simulink model "PWMGenerator"  (R2017a)
settings: Solver=VariableStepAuto  StartTime=0.0  StopTime=2000000  RelTol=1e-3
libraries: hdlsllib x15, simulink x5
settings Model: Creator=Ryan Corkery  LastModifiedBy=nguyen.se
settings OptimizationCC: BlockReduction=off  ConditionallyExecuteInputs=off  DefaultParameterBehavior=Inlined
settings DebuggingCC: AlgebraicLoopMsg=error
settings HardwareCC: ProdBitPerPointer=32  ProdBitPerSizeT=32  ProdBitPerPtrDiffT=32  ProdLargestAtomicFloat=None  ProdIntDivRoundTo=Undefined  ProdEndianess=Unspecified  ProdWordSize=32  ProdHWDeviceType=ASIC/FPGA->ASIC/FPGA  ProdEqTarget=off

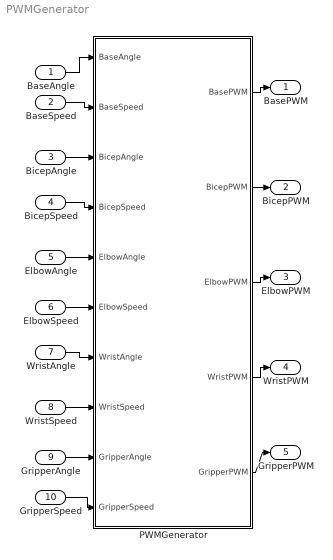
== system PWMGenerator ==
  BaseAngle : Inport  OutDataTypeStr=uint8
  BaseSpeed : Inport  Port=2  OutDataTypeStr=uint8
  BicepAngle : Inport  Port=3  OutDataTypeStr=uint8
  BicepSpeed : Inport  Port=4  OutDataTypeStr=uint8
  ElbowAngle : Inport  Port=5  OutDataTypeStr=uint8
  ElbowSpeed : Inport  Port=6  OutDataTypeStr=uint8
  WristAngle : Inport  Port=7  OutDataTypeStr=uint8
  WristSpeed : Inport  Port=8  OutDataTypeStr=uint8
  GripperAngle : Inport  Port=9  OutDataTypeStr=uint8
  GripperSpeed : Inport  Port=10  OutDataTypeStr=uint8
  PWMGenerator : Subsystem
  BasePWM : Outport  OutDataTypeStr=boolean
  BicepPWM : Outport  Port=2  OutDataTypeStr=boolean
  ElbowPWM : Outport  Port=3  OutDataTypeStr=boolean
  WristPWM : Outport  Port=4  OutDataTypeStr=boolean
  GripperPWM : Outport  Port=5  OutDataTypeStr=boolean
  wires:
  BaseAngle/1 -> PWMGenerator/1(BaseAngle)
  BaseSpeed/1 -> PWMGenerator/2(BaseSpeed)
  BicepAngle/1 -> PWMGenerator/3(BicepAngle)
  BicepSpeed/1 -> PWMGenerator/4(BicepSpeed)
  ElbowAngle/1 -> PWMGenerator/5(ElbowAngle)
  ElbowSpeed/1 -> PWMGenerator/6(ElbowSpeed)
  WristAngle/1 -> PWMGenerator/7(WristAngle)
  WristSpeed/1 -> PWMGenerator/8(WristSpeed)
  GripperAngle/1 -> PWMGenerator/9(GripperAngle)
  GripperSpeed/1 -> PWMGenerator/10(GripperSpeed)
  PWMGenerator/1(BasePWM) -> BasePWM/1
  PWMGenerator/2(BicepPWM) -> BicepPWM/1
  PWMGenerator/3(ElbowPWM) -> ElbowPWM/1
  PWMGenerator/4(WristPWM) -> WristPWM/1
  PWMGenerator/5(GripperPWM) -> GripperPWM/1

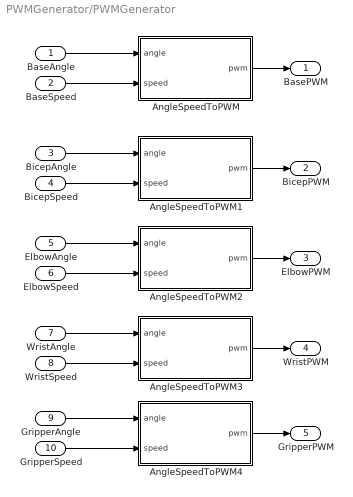
== system PWMGenerator/PWMGenerator ==
  BaseAngle : Inport  OutDataTypeStr=uint8
  BaseSpeed : Inport  Port=2  OutDataTypeStr=uint8
  BicepAngle : Inport  Port=3  OutDataTypeStr=uint8
  BicepSpeed : Inport  Port=4  OutDataTypeStr=uint8
  ElbowAngle : Inport  Port=5  OutDataTypeStr=uint8
  ElbowSpeed : Inport  Port=6  OutDataTypeStr=uint8
  WristAngle : Inport  Port=7  OutDataTypeStr=uint8
  WristSpeed : Inport  Port=8  OutDataTypeStr=uint8
  GripperAngle : Inport  Port=9  OutDataTypeStr=uint8
  GripperSpeed : Inport  Port=10  OutDataTypeStr=uint8
  AngleSpeedToPWM : Subsystem
  AngleSpeedToPWM1 : Subsystem
  AngleSpeedToPWM2 : Subsystem
  AngleSpeedToPWM3 : Subsystem
  AngleSpeedToPWM4 : Subsystem
  BasePWM : Outport  OutDataTypeStr=boolean
  BicepPWM : Outport  Port=2  OutDataTypeStr=boolean
  ElbowPWM : Outport  Port=3  OutDataTypeStr=boolean
  WristPWM : Outport  Port=4  OutDataTypeStr=boolean
  GripperPWM : Outport  Port=5  OutDataTypeStr=boolean
  wires:
  WristAngle/1 -> AngleSpeedToPWM3/1(angle)
  BaseAngle/1 -> AngleSpeedToPWM/1(angle)
  GripperSpeed/1 -> AngleSpeedToPWM4/2("speed ")
  WristSpeed/1 -> AngleSpeedToPWM3/2("speed ")
  GripperAngle/1 -> AngleSpeedToPWM4/1(angle)
  ElbowSpeed/1 -> AngleSpeedToPWM2/2("speed ")
  AngleSpeedToPWM/1(pwm) -> BasePWM/1
  AngleSpeedToPWM1/1(pwm) -> BicepPWM/1
  AngleSpeedToPWM2/1(pwm) -> ElbowPWM/1
  AngleSpeedToPWM3/1(pwm) -> WristPWM/1
  AngleSpeedToPWM4/1(pwm) -> GripperPWM/1
  BicepAngle/1 -> AngleSpeedToPWM1/1(angle)
  ElbowAngle/1 -> AngleSpeedToPWM2/1(angle)
  BicepSpeed/1 -> AngleSpeedToPWM1/2("speed ")
  BaseSpeed/1 -> AngleSpeedToPWM/2("speed ")

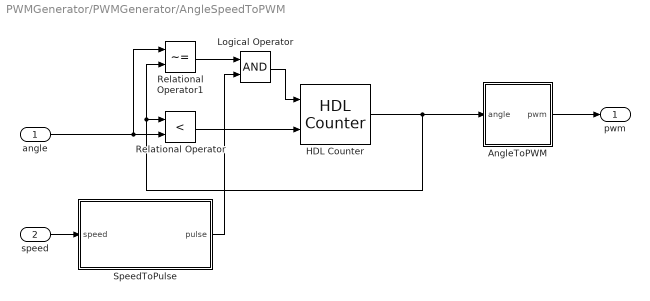
== system PWMGenerator/PWMGenerator/AngleSpeedToPWM ==
  angle : Inport  OutDataTypeStr=uint8
  "speed " : Inport  Port=2  OutDataTypeStr=uint8
  AngleToPWM : Subsystem
  HDL Counter : hdlsllib/HDL Operations/HDL Counter  CountType=Count limited  CountInit=90  CountStep=1  CountMax=180  CountFromType=Specify  CountFrom=0  CountResetPort=off  CountLoadPort=off  CountEnbPort=on  CountDirPort=on  CountDataType=Unsigned  CountWordLen=8  CountFracLen=0  CountSampTime=1
      settings: SourceProductName=HDL Coder  SourceProductBaseCode=HD
  Logical Operator : Logic  AllPortsSameDT=off  OutDataTypeStr=boolean
  Relational Operator : RelationalOperator  Operator=<  OutDataTypeStr=boolean  RndMeth=Simplest
  Relational Operator1 : RelationalOperator  Operator=~=  OutDataTypeStr=boolean  RndMeth=Simplest
  SpeedToPulse : Subsystem
  pwm : Outport  OutDataTypeStr=boolean
  wires:
  Relational Operator1/1 -> Logical Operator/1
  AngleToPWM/1(pwm) -> pwm/1
  HDL Counter/1 -> AngleToPWM/1("angle "), Relational Operator1/2, Relational Operator/1
  SpeedToPulse/1(pulse) -> Logical Operator/2
  Relational Operator/1 -> HDL Counter/2
  angle/1 -> Relational Operator1/1, Relational Operator/2
  Logical Operator/1 -> HDL Counter/1
  "speed "/1 -> SpeedToPulse/1(speed)

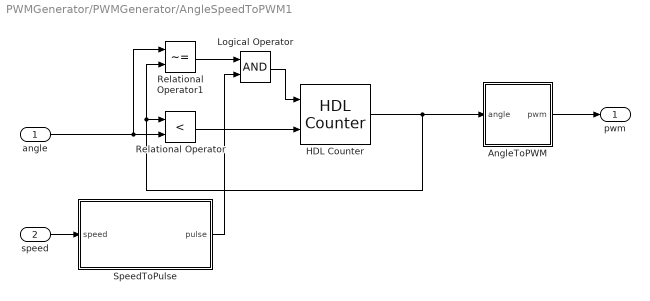
== system PWMGenerator/PWMGenerator/AngleSpeedToPWM1 ==
  angle : Inport  OutDataTypeStr=uint8
  "speed " : Inport  Port=2  OutDataTypeStr=uint8
  AngleToPWM : Subsystem
  HDL Counter : hdlsllib/HDL Operations/HDL Counter  CountType=Count limited  CountInit=90  CountStep=1  CountMax=180  CountFromType=Specify  CountFrom=0  CountResetPort=off  CountLoadPort=off  CountEnbPort=on  CountDirPort=on  CountDataType=Unsigned  CountWordLen=8  CountFracLen=0  CountSampTime=1
      settings: SourceProductName=HDL Coder  SourceProductBaseCode=HD
  Logical Operator : Logic  AllPortsSameDT=off  OutDataTypeStr=boolean
  Relational Operator : RelationalOperator  Operator=<  OutDataTypeStr=boolean  RndMeth=Simplest
  Relational Operator1 : RelationalOperator  Operator=~=  OutDataTypeStr=boolean  RndMeth=Simplest
  SpeedToPulse : Subsystem
  pwm : Outport  OutDataTypeStr=boolean
  wires:
  Relational Operator1/1 -> Logical Operator/1
  AngleToPWM/1(pwm) -> pwm/1
  HDL Counter/1 -> AngleToPWM/1("angle "), Relational Operator1/2, Relational Operator/1
  SpeedToPulse/1(pulse) -> Logical Operator/2
  Relational Operator/1 -> HDL Counter/2
  angle/1 -> Relational Operator1/1, Relational Operator/2
  Logical Operator/1 -> HDL Counter/1
  "speed "/1 -> SpeedToPulse/1(speed)

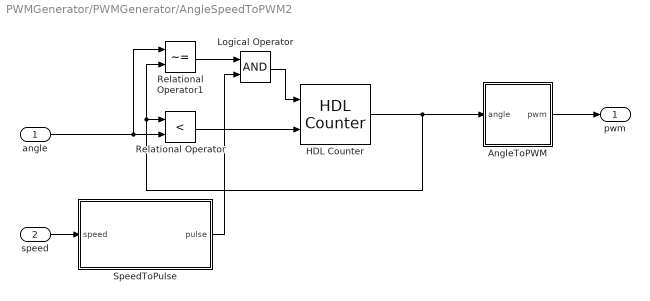
== system PWMGenerator/PWMGenerator/AngleSpeedToPWM2 ==
  angle : Inport  OutDataTypeStr=uint8
  "speed " : Inport  Port=2  OutDataTypeStr=uint8
  AngleToPWM : Subsystem
  HDL Counter : hdlsllib/HDL Operations/HDL Counter  CountType=Count limited  CountInit=90  CountStep=1  CountMax=180  CountFromType=Specify  CountFrom=0  CountResetPort=off  CountLoadPort=off  CountEnbPort=on  CountDirPort=on  CountDataType=Unsigned  CountWordLen=8  CountFracLen=0  CountSampTime=1
      settings: SourceProductName=HDL Coder  SourceProductBaseCode=HD
  Logical Operator : Logic  AllPortsSameDT=off  OutDataTypeStr=boolean
  Relational Operator : RelationalOperator  Operator=<  OutDataTypeStr=boolean  RndMeth=Simplest
  Relational Operator1 : RelationalOperator  Operator=~=  OutDataTypeStr=boolean  RndMeth=Simplest
  SpeedToPulse : Subsystem
  pwm : Outport  OutDataTypeStr=boolean
  wires:
  Relational Operator1/1 -> Logical Operator/1
  AngleToPWM/1(pwm) -> pwm/1
  HDL Counter/1 -> AngleToPWM/1("angle "), Relational Operator1/2, Relational Operator/1
  SpeedToPulse/1(pulse) -> Logical Operator/2
  Relational Operator/1 -> HDL Counter/2
  angle/1 -> Relational Operator1/1, Relational Operator/2
  Logical Operator/1 -> HDL Counter/1
  "speed "/1 -> SpeedToPulse/1(speed)

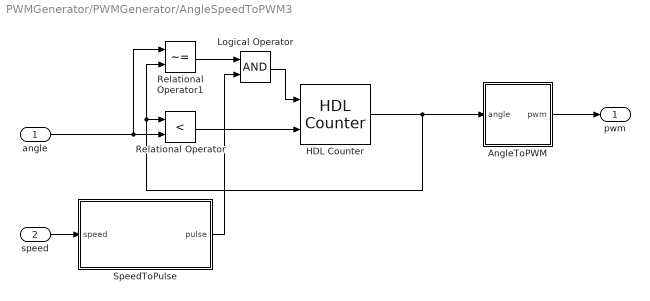
== system PWMGenerator/PWMGenerator/AngleSpeedToPWM3 ==
  angle : Inport  OutDataTypeStr=uint8
  "speed " : Inport  Port=2  OutDataTypeStr=uint8
  AngleToPWM : Subsystem
  HDL Counter : hdlsllib/HDL Operations/HDL Counter  CountType=Count limited  CountInit=90  CountStep=1  CountMax=180  CountFromType=Specify  CountFrom=0  CountResetPort=off  CountLoadPort=off  CountEnbPort=on  CountDirPort=on  CountDataType=Unsigned  CountWordLen=8  CountFracLen=0  CountSampTime=1
      settings: SourceProductName=HDL Coder  SourceProductBaseCode=HD
  Logical Operator : Logic  AllPortsSameDT=off  OutDataTypeStr=boolean
  Relational Operator : RelationalOperator  Operator=<  OutDataTypeStr=boolean  RndMeth=Simplest
  Relational Operator1 : RelationalOperator  Operator=~=  OutDataTypeStr=boolean  RndMeth=Simplest
  SpeedToPulse : Subsystem
  pwm : Outport  OutDataTypeStr=boolean
  wires:
  Relational Operator1/1 -> Logical Operator/1
  AngleToPWM/1(pwm) -> pwm/1
  HDL Counter/1 -> AngleToPWM/1("angle "), Relational Operator1/2, Relational Operator/1
  SpeedToPulse/1(pulse) -> Logical Operator/2
  Relational Operator/1 -> HDL Counter/2
  angle/1 -> Relational Operator1/1, Relational Operator/2
  Logical Operator/1 -> HDL Counter/1
  "speed "/1 -> SpeedToPulse/1(speed)

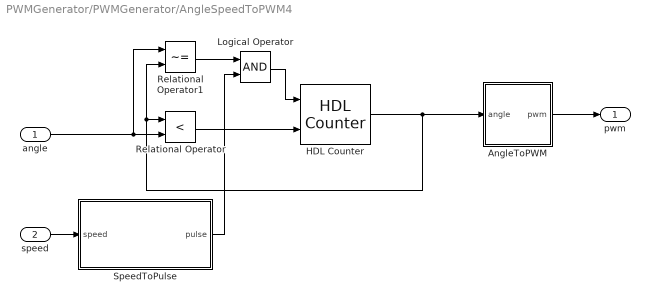
== system PWMGenerator/PWMGenerator/AngleSpeedToPWM4 ==
  angle : Inport  OutDataTypeStr=uint8
  "speed " : Inport  Port=2  OutDataTypeStr=uint8
  AngleToPWM : Subsystem
  HDL Counter : hdlsllib/HDL Operations/HDL Counter  CountType=Count limited  CountInit=90  CountStep=1  CountMax=180  CountFromType=Specify  CountFrom=0  CountResetPort=off  CountLoadPort=off  CountEnbPort=on  CountDirPort=on  CountDataType=Unsigned  CountWordLen=8  CountFracLen=0  CountSampTime=1
      settings: SourceProductName=HDL Coder  SourceProductBaseCode=HD
  Logical Operator : Logic  AllPortsSameDT=off  OutDataTypeStr=boolean
  Relational Operator : RelationalOperator  Operator=<  OutDataTypeStr=boolean  RndMeth=Simplest
  Relational Operator1 : RelationalOperator  Operator=~=  OutDataTypeStr=boolean  RndMeth=Simplest
  SpeedToPulse : Subsystem
  pwm : Outport  OutDataTypeStr=boolean
  wires:
  Relational Operator1/1 -> Logical Operator/1
  AngleToPWM/1(pwm) -> pwm/1
  HDL Counter/1 -> AngleToPWM/1("angle "), Relational Operator1/2, Relational Operator/1
  SpeedToPulse/1(pulse) -> Logical Operator/2
  Relational Operator/1 -> HDL Counter/2
  angle/1 -> Relational Operator1/1, Relational Operator/2
  Logical Operator/1 -> HDL Counter/1
  "speed "/1 -> SpeedToPulse/1(speed)

== system PWMGenerator/PWMGenerator/AngleSpeedToPWM/AngleToPWM ==
  "angle " : Inport  OutDataTypeStr=uint8
  Angle to PWM : Subsystem
  pwm : Outport
  wires:
  "angle "/1 -> Angle to PWM/1("angle ")
  Angle to PWM/1(pwm) -> pwm/1

== system PWMGenerator/PWMGenerator/AngleSpeedToPWM/SpeedToPulse ==
  speed : Inport  OutDataTypeStr=uint8
  Compare To Constant : simulink/Logic and Bit Operations/Compare To Constant  relop===  const=0  OutDataTypeStr=boolean
  Constant : Constant  Value=50000000  OutDataTypeStr=uint32  SampleTime=1
  Divide : Product  Inputs=*/  SaturateOnIntegerOverflow=on  RndMeth=Zero
  HDL Counter : hdlsllib/HDL Operations/HDL Counter  CountType=Free running  CountInit=0  CountStep=1  CountMax=25  CountFromType=Initial value  CountFrom=0  CountResetPort=on  CountLoadPort=off  CountEnbPort=off  CountDirPort=off  CountDataType=Unsigned  CountWordLen=32  CountFracLen=0  CountSampTime=1
      settings: SourceProductName=HDL Coder  SourceProductBaseCode=HD
  Relational Operator : RelationalOperator  Operator=<=  OutDataTypeStr=boolean  RndMeth=Nearest
  pulse : Outport
  wires:
  Divide/1 -> Relational Operator/1
  Compare To Constant/1 -> pulse/1
  HDL Counter/1 -> Relational Operator/2, Compare To Constant/1
  Relational Operator/1 -> HDL Counter/1
  Constant/1 -> Divide/1
  speed/1 -> Divide/2

== system PWMGenerator/PWMGenerator/AngleSpeedToPWM1/AngleToPWM ==
  "angle " : Inport  OutDataTypeStr=uint8
  Angle to PWM : Subsystem
  pwm : Outport
  wires:
  "angle "/1 -> Angle to PWM/1("angle ")
  Angle to PWM/1(pwm) -> pwm/1

== system PWMGenerator/PWMGenerator/AngleSpeedToPWM1/SpeedToPulse ==
  speed : Inport  OutDataTypeStr=uint8
  Compare To Constant : simulink/Logic and Bit Operations/Compare To Constant  relop===  const=0  OutDataTypeStr=boolean
  Constant : Constant  Value=50000000  OutDataTypeStr=uint32  SampleTime=1
  Divide : Product  Inputs=*/  SaturateOnIntegerOverflow=on  RndMeth=Zero
  HDL Counter : hdlsllib/HDL Operations/HDL Counter  CountType=Free running  CountInit=0  CountStep=1  CountMax=25  CountFromType=Initial value  CountFrom=0  CountResetPort=on  CountLoadPort=off  CountEnbPort=off  CountDirPort=off  CountDataType=Unsigned  CountWordLen=32  CountFracLen=0  CountSampTime=1
      settings: SourceProductName=HDL Coder  SourceProductBaseCode=HD
  Relational Operator : RelationalOperator  Operator=<=  OutDataTypeStr=boolean  RndMeth=Nearest
  pulse : Outport
  wires:
  Divide/1 -> Relational Operator/1
  Compare To Constant/1 -> pulse/1
  HDL Counter/1 -> Relational Operator/2, Compare To Constant/1
  Relational Operator/1 -> HDL Counter/1
  Constant/1 -> Divide/1
  speed/1 -> Divide/2

== system PWMGenerator/PWMGenerator/AngleSpeedToPWM2/AngleToPWM ==
  "angle " : Inport  OutDataTypeStr=uint8
  Angle to PWM : Subsystem
  pwm : Outport
  wires:
  "angle "/1 -> Angle to PWM/1("angle ")
  Angle to PWM/1(pwm) -> pwm/1

== system PWMGenerator/PWMGenerator/AngleSpeedToPWM2/SpeedToPulse ==
  speed : Inport  OutDataTypeStr=uint8
  Compare To Constant : simulink/Logic and Bit Operations/Compare To Constant  relop===  const=0  OutDataTypeStr=boolean
  Constant : Constant  Value=50000000  OutDataTypeStr=uint32  SampleTime=1
  Divide : Product  Inputs=*/  SaturateOnIntegerOverflow=on  RndMeth=Zero
  HDL Counter : hdlsllib/HDL Operations/HDL Counter  CountType=Free running  CountInit=0  CountStep=1  CountMax=25  CountFromType=Initial value  CountFrom=0  CountResetPort=on  CountLoadPort=off  CountEnbPort=off  CountDirPort=off  CountDataType=Unsigned  CountWordLen=32  CountFracLen=0  CountSampTime=1
      settings: SourceProductName=HDL Coder  SourceProductBaseCode=HD
  Relational Operator : RelationalOperator  Operator=<=  OutDataTypeStr=boolean  RndMeth=Nearest
  pulse : Outport
  wires:
  Divide/1 -> Relational Operator/1
  Compare To Constant/1 -> pulse/1
  HDL Counter/1 -> Relational Operator/2, Compare To Constant/1
  Relational Operator/1 -> HDL Counter/1
  Constant/1 -> Divide/1
  speed/1 -> Divide/2

== system PWMGenerator/PWMGenerator/AngleSpeedToPWM3/AngleToPWM ==
  "angle " : Inport  OutDataTypeStr=uint8
  Angle to PWM : Subsystem
  pwm : Outport
  wires:
  "angle "/1 -> Angle to PWM/1("angle ")
  Angle to PWM/1(pwm) -> pwm/1

== system PWMGenerator/PWMGenerator/AngleSpeedToPWM3/SpeedToPulse ==
  speed : Inport  OutDataTypeStr=uint8
  Compare To Constant : simulink/Logic and Bit Operations/Compare To Constant  relop===  const=0  OutDataTypeStr=boolean
  Constant : Constant  Value=50000000  OutDataTypeStr=uint32  SampleTime=1
  Divide : Product  Inputs=*/  SaturateOnIntegerOverflow=on  RndMeth=Zero
  HDL Counter : hdlsllib/HDL Operations/HDL Counter  CountType=Free running  CountInit=0  CountStep=1  CountMax=25  CountFromType=Initial value  CountFrom=0  CountResetPort=on  CountLoadPort=off  CountEnbPort=off  CountDirPort=off  CountDataType=Unsigned  CountWordLen=32  CountFracLen=0  CountSampTime=1
      settings: SourceProductName=HDL Coder  SourceProductBaseCode=HD
  Relational Operator : RelationalOperator  Operator=<=  OutDataTypeStr=boolean  RndMeth=Nearest
  pulse : Outport
  wires:
  Divide/1 -> Relational Operator/1
  Compare To Constant/1 -> pulse/1
  HDL Counter/1 -> Relational Operator/2, Compare To Constant/1
  Relational Operator/1 -> HDL Counter/1
  Constant/1 -> Divide/1
  speed/1 -> Divide/2

== system PWMGenerator/PWMGenerator/AngleSpeedToPWM4/AngleToPWM ==
  "angle " : Inport  OutDataTypeStr=uint8
  Angle to PWM : Subsystem
  pwm : Outport
  wires:
  "angle "/1 -> Angle to PWM/1("angle ")
  Angle to PWM/1(pwm) -> pwm/1

== system PWMGenerator/PWMGenerator/AngleSpeedToPWM4/SpeedToPulse ==
  speed : Inport  OutDataTypeStr=uint8
  Compare To Constant : simulink/Logic and Bit Operations/Compare To Constant  relop===  const=0  OutDataTypeStr=boolean
  Constant : Constant  Value=50000000  OutDataTypeStr=uint32  SampleTime=1
  Divide : Product  Inputs=*/  SaturateOnIntegerOverflow=on  RndMeth=Zero
  HDL Counter : hdlsllib/HDL Operations/HDL Counter  CountType=Free running  CountInit=0  CountStep=1  CountMax=25  CountFromType=Initial value  CountFrom=0  CountResetPort=on  CountLoadPort=off  CountEnbPort=off  CountDirPort=off  CountDataType=Unsigned  CountWordLen=32  CountFracLen=0  CountSampTime=1
      settings: SourceProductName=HDL Coder  SourceProductBaseCode=HD
  Relational Operator : RelationalOperator  Operator=<=  OutDataTypeStr=boolean  RndMeth=Nearest
  pulse : Outport
  wires:
  Divide/1 -> Relational Operator/1
  Compare To Constant/1 -> pulse/1
  HDL Counter/1 -> Relational Operator/2, Compare To Constant/1
  Relational Operator/1 -> HDL Counter/1
  Constant/1 -> Divide/1
  speed/1 -> Divide/2

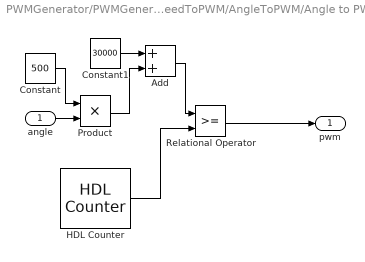
== system PWMGenerator/PWMGenerator/AngleSpeedToPWM/AngleToPWM/Angle to PWM ==
  "angle " : Inport  OutDataTypeStr=uint8
  Add : Sum
  Constant : Constant  Value=500  OutDataTypeStr=uint32  SampleTime=1
  Constant1 : Constant  Value=30000  OutDataTypeStr=uint32  SampleTime=1
  HDL Counter : hdlsllib/HDL Operations/HDL Counter  CountType=Count limited  CountInit=0  CountStep=1  CountMax=1000000  CountFromType=Initial value  CountFrom=0  CountResetPort=off  CountLoadPort=off  CountEnbPort=off  CountDirPort=off  CountDataType=Unsigned  CountWordLen=32  CountFracLen=0  CountSampTime=1
      settings: SourceProductName=HDL Coder  SourceProductBaseCode=HD
  Product : Product
  Relational Operator : RelationalOperator  OutDataTypeStr=boolean  RndMeth=Simplest
  pwm : Outport
  wires:
  HDL Counter/1 -> Relational Operator/2
  Relational Operator/1 -> pwm/1
  Product/1 -> Add/2
  Constant/1 -> Product/1
  "angle "/1 -> Product/2
  Constant1/1 -> Add/1
  Add/1 -> Relational Operator/1

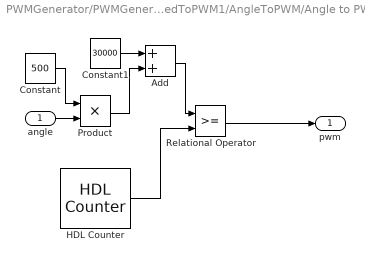
== system PWMGenerator/PWMGenerator/AngleSpeedToPWM1/AngleToPWM/Angle to PWM ==
  "angle " : Inport  OutDataTypeStr=uint8
  Add : Sum
  Constant : Constant  Value=500  OutDataTypeStr=uint32  SampleTime=1
  Constant1 : Constant  Value=30000  OutDataTypeStr=uint32  SampleTime=1
  HDL Counter : hdlsllib/HDL Operations/HDL Counter  CountType=Count limited  CountInit=0  CountStep=1  CountMax=1000000  CountFromType=Initial value  CountFrom=0  CountResetPort=off  CountLoadPort=off  CountEnbPort=off  CountDirPort=off  CountDataType=Unsigned  CountWordLen=32  CountFracLen=0  CountSampTime=1
      settings: SourceProductName=HDL Coder  SourceProductBaseCode=HD
  Product : Product
  Relational Operator : RelationalOperator  OutDataTypeStr=boolean  RndMeth=Simplest
  pwm : Outport
  wires:
  HDL Counter/1 -> Relational Operator/2
  Relational Operator/1 -> pwm/1
  Product/1 -> Add/2
  Constant/1 -> Product/1
  "angle "/1 -> Product/2
  Constant1/1 -> Add/1
  Add/1 -> Relational Operator/1

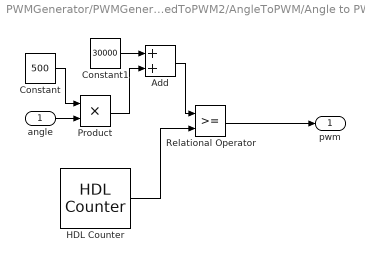
== system PWMGenerator/PWMGenerator/AngleSpeedToPWM2/AngleToPWM/Angle to PWM ==
  "angle " : Inport  OutDataTypeStr=uint8
  Add : Sum
  Constant : Constant  Value=500  OutDataTypeStr=uint32  SampleTime=1
  Constant1 : Constant  Value=30000  OutDataTypeStr=uint32  SampleTime=1
  HDL Counter : hdlsllib/HDL Operations/HDL Counter  CountType=Count limited  CountInit=0  CountStep=1  CountMax=1000000  CountFromType=Initial value  CountFrom=0  CountResetPort=off  CountLoadPort=off  CountEnbPort=off  CountDirPort=off  CountDataType=Unsigned  CountWordLen=32  CountFracLen=0  CountSampTime=1
      settings: SourceProductName=HDL Coder  SourceProductBaseCode=HD
  Product : Product
  Relational Operator : RelationalOperator  OutDataTypeStr=boolean  RndMeth=Simplest
  pwm : Outport
  wires:
  HDL Counter/1 -> Relational Operator/2
  Relational Operator/1 -> pwm/1
  Product/1 -> Add/2
  Constant/1 -> Product/1
  "angle "/1 -> Product/2
  Constant1/1 -> Add/1
  Add/1 -> Relational Operator/1

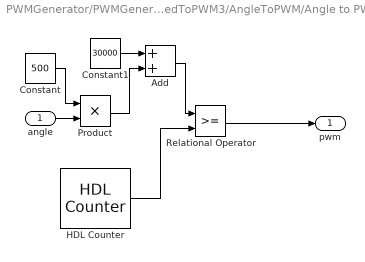
== system PWMGenerator/PWMGenerator/AngleSpeedToPWM3/AngleToPWM/Angle to PWM ==
  "angle " : Inport  OutDataTypeStr=uint8
  Add : Sum
  Constant : Constant  Value=500  OutDataTypeStr=uint32  SampleTime=1
  Constant1 : Constant  Value=30000  OutDataTypeStr=uint32  SampleTime=1
  HDL Counter : hdlsllib/HDL Operations/HDL Counter  CountType=Count limited  CountInit=0  CountStep=1  CountMax=1000000  CountFromType=Initial value  CountFrom=0  CountResetPort=off  CountLoadPort=off  CountEnbPort=off  CountDirPort=off  CountDataType=Unsigned  CountWordLen=32  CountFracLen=0  CountSampTime=1
      settings: SourceProductName=HDL Coder  SourceProductBaseCode=HD
  Product : Product
  Relational Operator : RelationalOperator  OutDataTypeStr=boolean  RndMeth=Simplest
  pwm : Outport
  wires:
  HDL Counter/1 -> Relational Operator/2
  Relational Operator/1 -> pwm/1
  Product/1 -> Add/2
  Constant/1 -> Product/1
  "angle "/1 -> Product/2
  Constant1/1 -> Add/1
  Add/1 -> Relational Operator/1

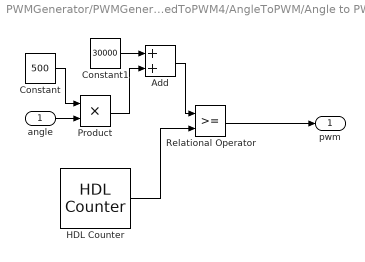
== system PWMGenerator/PWMGenerator/AngleSpeedToPWM4/AngleToPWM/Angle to PWM ==
  "angle " : Inport  OutDataTypeStr=uint8
  Add : Sum
  Constant : Constant  Value=500  OutDataTypeStr=uint32  SampleTime=1
  Constant1 : Constant  Value=30000  OutDataTypeStr=uint32  SampleTime=1
  HDL Counter : hdlsllib/HDL Operations/HDL Counter  CountType=Count limited  CountInit=0  CountStep=1  CountMax=1000000  CountFromType=Initial value  CountFrom=0  CountResetPort=off  CountLoadPort=off  CountEnbPort=off  CountDirPort=off  CountDataType=Unsigned  CountWordLen=32  CountFracLen=0  CountSampTime=1
      settings: SourceProductName=HDL Coder  SourceProductBaseCode=HD
  Product : Product
  Relational Operator : RelationalOperator  OutDataTypeStr=boolean  RndMeth=Simplest
  pwm : Outport
  wires:
  HDL Counter/1 -> Relational Operator/2
  Relational Operator/1 -> pwm/1
  Product/1 -> Add/2
  Constant/1 -> Product/1
  "angle "/1 -> Product/2
  Constant1/1 -> Add/1
  Add/1 -> Relational Operator/1
